simulink library "Sanu_Lib"  (R2025b)
settings: Solver=VariableStepAuto  StartTime=0.0  StopTime=10.0  RelTol=1e-3
libraries: simulink x16
settings Model: Creator=2503-00091  LastModifiedBy=2503-00091

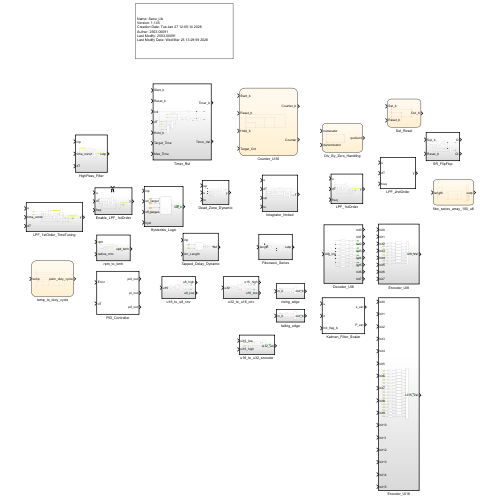
[thumbnail: Simulink's stored preview of the top-level diagram]
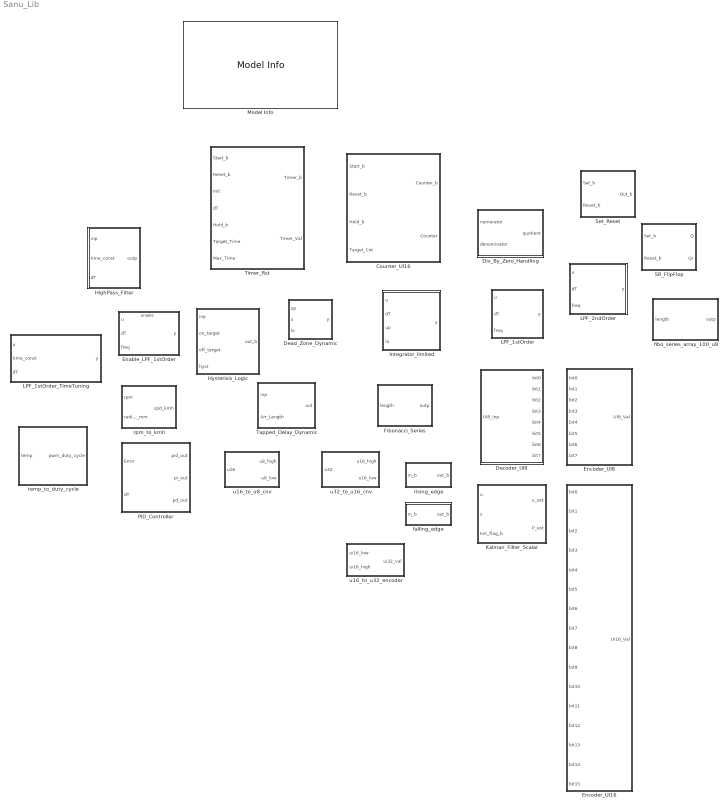
== system Sanu_Lib ==
  Counter_UI16 : Stateflow chart  TreatAsAtomicUnit=on  RTWFcnName=Counter_UI16  RTWFileName=Counter_UI16
      settings: RTWSystemCode=Reusable function  RTWFcnNameOpts=User specified  RTWFileNameOpts=User specified
  Dead_Zone_Dynamic : Subsystem  TreatAsAtomicUnit=on  RTWFcnName=Dead_Zone_Dynamic  RTWFileName=Dead_Zone_Dynamic
      settings: RTWFcnNameOpts=User specified  RTWFileNameOpts=User specified
  Decoder_UI8 : Subsystem  TreatAsAtomicUnit=on  RTWFcnName=Decoder_UI8  RTWFileName=Decoder_UI8
      settings: RTWFcnNameOpts=User specified  RTWFileNameOpts=User specified
  Div_By_Zero_Handling : Stateflow chart  TreatAsAtomicUnit=on  RTWFcnName=Div_By_Zero_Handling  RTWFileName=Div_By_Zero_Handling
      settings: RTWSystemCode=Reusable function  RTWFcnNameOpts=User specified  RTWFileNameOpts=User specified
  Enable_LPF_1stOrder : Subsystem  RTWFcnName=Enable_LPF_1stOrder  RTWFileName=Enable_LPF_1stOrder
      settings: RTWFcnNameOpts=User specified  RTWFileNameOpts=User specified
  Encoder_UI16 : Subsystem  TreatAsAtomicUnit=on  RTWFcnName=Encoder_UI16  RTWFileName=Encoder_UI16
      settings: RTWFcnNameOpts=User specified  RTWFileNameOpts=User specified
  Encoder_UI8 : Subsystem  TreatAsAtomicUnit=on  RTWFcnName=Encoder_UI8  RTWFileName=Encoder_UI8
      settings: RTWFcnNameOpts=User specified  RTWFileNameOpts=User specified
  Fibonacci_Series : Subsystem  TreatAsAtomicUnit=on  RTWFcnName=fibonacci_series_U8  RTWFileName=fibonacci_series_U8
      settings: RTWFcnNameOpts=User specified  RTWFileNameOpts=User specified
  HighPass_Filter : Subsystem  TreatAsAtomicUnit=on  RTWFcnName=HighPass_Filter  RTWFileName=HighPass_Filter
      settings: RTWFcnNameOpts=User specified  RTWFileNameOpts=User specified
  Hysterisis_Logic : Subsystem  TreatAsAtomicUnit=on  RTWFcnName=Hysterisis_Logic  RTWFileName=Hysterisis_Logic
      settings: RTWFcnNameOpts=User specified  RTWFileNameOpts=User specified
  Integrator_limited : Subsystem  TreatAsAtomicUnit=on  RTWFcnName=Integrator_limited  RTWFileName=Integrator_limited
      settings: RTWFcnNameOpts=User specified  RTWFileNameOpts=User specified
  Kalman_Filter_Scalar : Subsystem  TreatAsAtomicUnit=on  RTWFcnName=Kalman_Filter_Scalar  RTWFileName=Kalman_Filter_Scalar  mask{A_Gain=1, B_Gain=0, H_Gain=1, Q_Gain=0.01, R_Gain=0.1, x_est_init=0, P_est_init=1}
      settings: RTWFcnNameOpts=User specified  RTWFileNameOpts=User specified
      mask TypeOptions A_Gain: A_Gain/Value
      mask TypeOptions B_Gain: B_Gain/Gain
      mask TypeOptions H_Gain: H_Gain/Value
      mask TypeOptions Q_Gain: Q_Const/Value
      mask TypeOptions R_Gain: R_Const/Value
      mask TypeOptions x_est_init: x_init/Value
      mask TypeOptions P_est_init: P_init/Value
  LPF_1stOrder : Subsystem  TreatAsAtomicUnit=on  RTWFcnName=LPF_1stOrder  RTWFileName=LPF_1stOrder
      settings: RTWFcnNameOpts=User specified  RTWFileNameOpts=User specified
  LPF_1stOrder_TimeTuning : Subsystem  TreatAsAtomicUnit=on  RTWFcnName=LPF_1stOrder_TimeTuning  RTWFileName=LPF_1stOrder_TimeTuning
      settings: RTWFcnNameOpts=User specified  RTWFileNameOpts=User specified
  LPF_2ndOrder : Subsystem  TreatAsAtomicUnit=on  RTWFcnName=LPF_2ndOrder  RTWFileName=LPF_2ndOrder  mask{Gain=1}
      mask prompts: Gain "Damping_Coefficient:"
      settings: RTWFcnNameOpts=User specified  RTWFileNameOpts=User specified
      mask TypeOptions Gain: damping_coeff/Gain
  Model Info : simulink/Model-Wide Utilities/Model Info  Frame=on  DisplayStringWithTags=|  HorizontalTextAlignment=Left  LeftAlignmentValue=0.02
      | Name: %<ModelName>
      | Version: %<ModelVersion>
      | Creation Date: %<Created>
      | Author: %<Creator>
      | Last Modify: %<LastModifiedBy>
      | Last Modify Date: %<LastModificationDate>
  PID_Controller : Subsystem  TreatAsAtomicUnit=on  RTWFcnName=PID_Controller  RTWFileName=PID_Controller  mask{P_Gain=1, I_Gain=1, D_Gain=0, N_Gain=100}
      mask prompts: N_Gain "Filter(N)_Coeff:"
      settings: RTWFcnNameOpts=User specified  RTWFileNameOpts=User specified
      mask TypeOptions P_Gain: P_Gain/Gain
      mask TypeOptions I_Gain: I_Gain/Gain
      mask TypeOptions D_Gain: D_Gain/Gain
      mask TypeOptions N_Gain: N_Coeff/Gain
  SR_FlipFlop : Subsystem  TreatAsAtomicUnit=on  RTWFcnName=SR_FlipFlop  RTWFileName=SR_FlipFlop
      settings: RTWFcnNameOpts=User specified  RTWFileNameOpts=User specified
  Set_Reset : Stateflow chart  TreatAsAtomicUnit=on  RTWFcnName=Set_Reset  RTWFileName=Set_Reset
      settings: RTWSystemCode=Reusable function  RTWFcnNameOpts=User specified  RTWFileNameOpts=User specified
  Tapped_Delay_Dynamic : Subsystem  TreatAsAtomicUnit=on  RTWFcnName=Tapped_Delay_Dynamic  RTWFileName=Tapped_Delay_Dynamic
      settings: RTWFcnNameOpts=User specified  RTWFileNameOpts=User specified
  Timer_Rst : Subsystem  TreatAsAtomicUnit=on  RTWFcnName=Timer_Rst  RTWFileName=Timer_Rst
      settings: RTWFcnNameOpts=User specified  RTWFileNameOpts=User specified
  falling_edge : Subsystem  TreatAsAtomicUnit=on  RTWFcnName=falling_edge  RTWFileName=falling_edge
      settings: RTWFcnNameOpts=User specified  RTWFileNameOpts=User specified
  fibo_series_array_100_u8 : Stateflow chart  TreatAsAtomicUnit=on  RTWFcnName=fibo_series_array_100_u8  RTWFileName=fibo_series_array_100_u8
      settings: RTWSystemCode=Reusable function  RTWFcnNameOpts=User specified  RTWFileNameOpts=User specified
  rising_edge : Subsystem  TreatAsAtomicUnit=on  RTWFcnName=rising_edge  RTWFileName=rising_edge
      settings: RTWFcnNameOpts=User specified  RTWFileNameOpts=User specified
  rpm_to_kmh : Subsystem  TreatAsAtomicUnit=on  RTWFcnName=rpm_to_kmph  RTWFileName=rpm_to_kmph
      settings: RTWFcnNameOpts=User specified  RTWFileNameOpts=User specified
  temp_to_duty_cycle : Stateflow chart  TreatAsAtomicUnit=on  RTWFcnName=temp_to_duty_cycle  RTWFileName=temp_to_duty_cycle
      settings: RTWSystemCode=Reusable function  RTWFcnNameOpts=User specified  RTWFileNameOpts=User specified
  u16_to_u32_encoder : Subsystem  TreatAsAtomicUnit=on  RTWFcnName=u16_to_u32_encoder  RTWFileName=u16_to_u32_encoder
      settings: RTWFcnNameOpts=User specified  RTWFileNameOpts=User specified
  u16_to_u8_cnv : Subsystem  TreatAsAtomicUnit=on  RTWFcnName=u16_to_u8  RTWFileName=u16_to_u8
      settings: RTWFcnNameOpts=User specified  RTWFileNameOpts=User specified
  u32_to_u16_cnv : Subsystem  TreatAsAtomicUnit=on  RTWFcnName=u32_to_u16  RTWFileName=u32_to_u16
      settings: RTWFcnNameOpts=User specified  RTWFileNameOpts=User specified

== system Sanu_Lib/Dead_Zone_Dynamic ==
  up : Inport
  u : Inport  Port=2
  lo : Inport  Port=3
  Relational Operator : RelationalOperator  OutDataTypeStr=boolean  RndMeth=Simplest  InputSameDT=off
  Relational Operator1 : RelationalOperator  Operator=>  OutDataTypeStr=boolean  RndMeth=Simplest  InputSameDT=off
  Subtract : Sum  Inputs=+-
  Switch : Switch  Criteria=u2 ~= 0  SaturateOnIntegerOverflow=off  InputSameDT=off
  Switch1 : Switch  Criteria=u2 ~= 0  SaturateOnIntegerOverflow=off  InputSameDT=off
  y : Outport
  wires:
  up/1 -> Relational Operator/2, Switch/1
  u/1 -> Subtract/1, Relational Operator/1, Switch1/1, Relational Operator1/1
  Relational Operator/1 -> Switch/2
  Relational Operator1/1 -> Switch1/2
  lo/1 -> Switch1/3, Relational Operator1/2
  Switch1/1 -> Switch/3
  Subtract/1 -> y/1
  Switch/1 -> Subtract/2

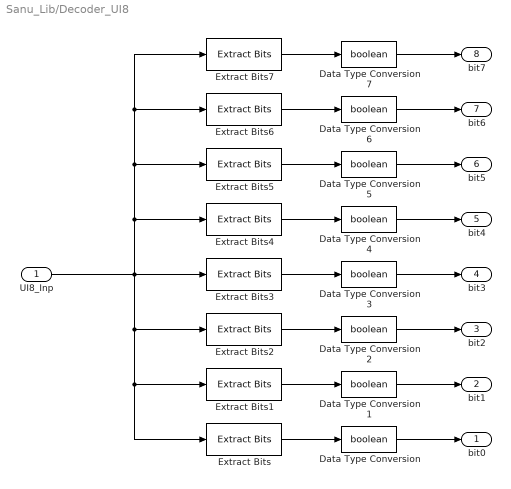
== system Sanu_Lib/Decoder_UI8 ==
  UI8_Inp : Inport  OutDataTypeStr=uint8
  Data Type Conversion{,1..7} (8 alike) : DataTypeConversion  OutDataTypeStr=boolean  SaturateOnIntegerOverflow=off  RndMeth=Floor
  Extract Bits : simulink/Logic and Bit Operations/Extract Bits  bitsToExtract=Range of bits  numBits=8  bitIdxRange=[0 0]  outScalingMode=Preserve fixed-point scaling
  Extract Bits1 : simulink/Logic and Bit Operations/Extract Bits  bitsToExtract=Range of bits  numBits=8  bitIdxRange=[1 1]  outScalingMode=Preserve fixed-point scaling
  Extract Bits2 : simulink/Logic and Bit Operations/Extract Bits  bitsToExtract=Range of bits  numBits=8  bitIdxRange=[2 2]  outScalingMode=Preserve fixed-point scaling
  Extract Bits3 : simulink/Logic and Bit Operations/Extract Bits  bitsToExtract=Range of bits  numBits=8  bitIdxRange=[3 3]  outScalingMode=Preserve fixed-point scaling
  Extract Bits4 : simulink/Logic and Bit Operations/Extract Bits  bitsToExtract=Range of bits  numBits=8  bitIdxRange=[4 4]  outScalingMode=Preserve fixed-point scaling
  Extract Bits5 : simulink/Logic and Bit Operations/Extract Bits  bitsToExtract=Range of bits  numBits=8  bitIdxRange=[5 5]  outScalingMode=Preserve fixed-point scaling
  Extract Bits6 : simulink/Logic and Bit Operations/Extract Bits  bitsToExtract=Range of bits  numBits=8  bitIdxRange=[6 6]  outScalingMode=Preserve fixed-point scaling
  Extract Bits7 : simulink/Logic and Bit Operations/Extract Bits  bitsToExtract=Range of bits  numBits=8  bitIdxRange=[7 7]  outScalingMode=Preserve fixed-point scaling
  bit0 : Outport
  bit1 : Outport  Port=2
  bit2 : Outport  Port=3
  bit3 : Outport  Port=4
  bit4 : Outport  Port=5
  bit5 : Outport  Port=6
  bit6 : Outport  Port=7
  bit7 : Outport  Port=8
  wires:
  UI8_Inp/1 -> Extract Bits5/1, Extract Bits6/1, Extract Bits7/1, Extract Bits4/1, Extract Bits3/1, Extract Bits2/1, Extract Bits1/1, Extract Bits/1
  Extract Bits/1 -> Data Type Conversion/1
  Data Type Conversion/1 -> bit0/1
  Data Type Conversion1/1 -> bit1/1
  Data Type Conversion3/1 -> bit3/1
  Data Type Conversion2/1 -> bit2/1
  Data Type Conversion4/1 -> bit4/1
  Data Type Conversion5/1 -> bit5/1
  Data Type Conversion7/1 -> bit7/1
  Data Type Conversion6/1 -> bit6/1
  Extract Bits1/1 -> Data Type Conversion1/1
  Extract Bits2/1 -> Data Type Conversion2/1
  Extract Bits3/1 -> Data Type Conversion3/1
  Extract Bits4/1 -> Data Type Conversion4/1
  Extract Bits5/1 -> Data Type Conversion5/1
  Extract Bits6/1 -> Data Type Conversion6/1
  Extract Bits7/1 -> Data Type Conversion7/1

== system Sanu_Lib/Enable_LPF_1stOrder ==
  note: y(t) = y(t-1) + (u(t) - y(t-1)) * dT * freq
  u : Inport
  dT : Inport  Port=2
  freq : Inport  Port=3
  Enable : EnablePort  StatesWhenEnabling=reset
  Product : Product
  Product1 : Product
  Substract : Sum  Inputs=+-
  delay_y : UnitDelay  SampleTime=-1  HasFrameUpgradeWarning=on
      settings: AttributesFormatString=Init: %<InitialCondition>
  lpf_out : Sum
  y : Outport
  wires:
  Product1/1 -> lpf_out/1
  freq/1 -> Product1/1
  lpf_out/1 -> delay_y/1, y/1
  u/1 -> Substract/1
  Product/1 -> Product1/2
  Substract/1 -> Product/2
  dT/1 -> Product/1
  delay_y/1 -> Substract/2, lpf_out/2

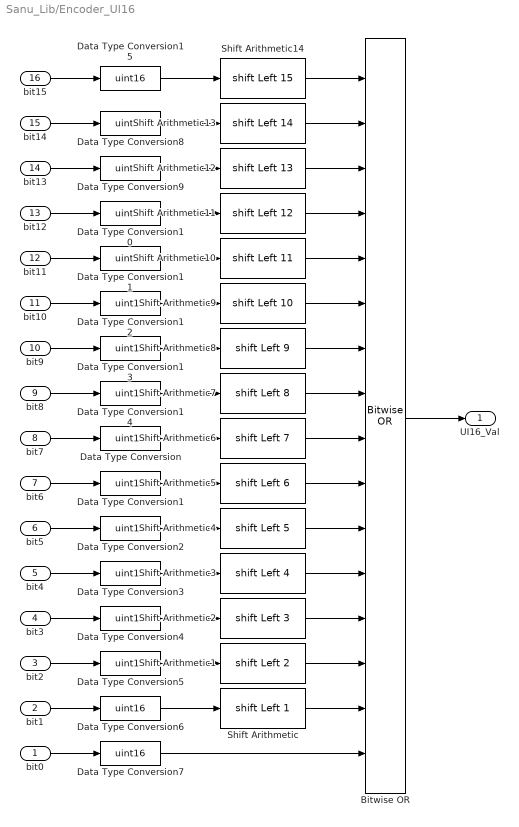
== system Sanu_Lib/Encoder_UI16 ==
  bit0 : Inport  OutDataTypeStr=boolean
  bit1 : Inport  Port=2  OutDataTypeStr=boolean
  bit2 : Inport  Port=3  OutDataTypeStr=boolean
  bit3 : Inport  Port=4  OutDataTypeStr=boolean
  bit4 : Inport  Port=5  OutDataTypeStr=boolean
  bit5 : Inport  Port=6  OutDataTypeStr=boolean
  bit6 : Inport  Port=7  OutDataTypeStr=boolean
  bit7 : Inport  Port=8  OutDataTypeStr=boolean
  bit8 : Inport  Port=9  OutDataTypeStr=boolean
  bit9 : Inport  Port=10  OutDataTypeStr=boolean
  bit10 : Inport  Port=11  OutDataTypeStr=boolean
  bit11 : Inport  Port=12  OutDataTypeStr=boolean
  bit12 : Inport  Port=13  OutDataTypeStr=boolean
  bit13 : Inport  Port=14  OutDataTypeStr=boolean
  bit14 : Inport  Port=15  OutDataTypeStr=boolean
  bit15 : Inport  Port=16  OutDataTypeStr=boolean
  Bitwise OR : simulink/Logic and Bit Operations/Bitwise Operator  logicop=OR  UseBitMask=off  NumInputPorts=16  BitMask=bin2dec('11011001')  BitMaskRealWorld=Stored Integer
      settings: LibrarySourceBlock=|
      | simulink/Quick Insert/Logic and Bit
      | Operations/Bitwise OR
  Data Type Conversion{,1..15} (16 alike) : DataTypeConversion  OutDataTypeStr=uint16  SaturateOnIntegerOverflow=off  RndMeth=Floor
  Shift Arithmetic : ArithShift  BitShiftNumber=1  BitShiftDirection=Left
  Shift Arithmetic1 : ArithShift  BitShiftNumber=2  BitShiftDirection=Left
  Shift Arithmetic10 : ArithShift  BitShiftNumber=11  BitShiftDirection=Left
  Shift Arithmetic11 : ArithShift  BitShiftNumber=12  BitShiftDirection=Left
  Shift Arithmetic12 : ArithShift  BitShiftNumber=13  BitShiftDirection=Left
  Shift Arithmetic13 : ArithShift  BitShiftNumber=14  BitShiftDirection=Left
  Shift Arithmetic14 : ArithShift  BitShiftNumber=15  BitShiftDirection=Left
  Shift Arithmetic2 : ArithShift  BitShiftNumber=3  BitShiftDirection=Left
  Shift Arithmetic3 : ArithShift  BitShiftNumber=4  BitShiftDirection=Left
  Shift Arithmetic4 : ArithShift  BitShiftNumber=5  BitShiftDirection=Left
  Shift Arithmetic5 : ArithShift  BitShiftNumber=6  BitShiftDirection=Left
  Shift Arithmetic6 : ArithShift  BitShiftNumber=7  BitShiftDirection=Left
  Shift Arithmetic7 : ArithShift  BitShiftNumber=8  BitShiftDirection=Left
  Shift Arithmetic8 : ArithShift  BitShiftNumber=9  BitShiftDirection=Left
  Shift Arithmetic9 : ArithShift  BitShiftNumber=10  BitShiftDirection=Left
  UI16_Val : Outport
  wires:
  bit7/1 -> Data Type Conversion/1
  bit2/1 -> Data Type Conversion5/1
  bit5/1 -> Data Type Conversion2/1
  Data Type Conversion1/1 -> Shift Arithmetic5/1
  Data Type Conversion2/1 -> Shift Arithmetic4/1
  Data Type Conversion4/1 -> Shift Arithmetic2/1
  bit0/1 -> Data Type Conversion7/1
  Data Type Conversion3/1 -> Shift Arithmetic3/1
  bit3/1 -> Data Type Conversion4/1
  Bitwise OR/1 -> UI16_Val/1
  Data Type Conversion6/1 -> Shift Arithmetic/1
  Data Type Conversion5/1 -> Shift Arithmetic1/1
  bit6/1 -> Data Type Conversion1/1
  Data Type Conversion/1 -> Shift Arithmetic6/1
  bit1/1 -> Data Type Conversion6/1
  bit4/1 -> Data Type Conversion3/1
  Shift Arithmetic1/1 -> Bitwise OR/14
  Shift Arithmetic/1 -> Bitwise OR/15
  Shift Arithmetic2/1 -> Bitwise OR/13
  Data Type Conversion7/1 -> Bitwise OR/16
  Shift Arithmetic3/1 -> Bitwise OR/12
  bit11/1 -> Data Type Conversion11/1
  bit8/1 -> Data Type Conversion14/1
  Data Type Conversion8/1 -> Shift Arithmetic13/1
  bit13/1 -> Data Type Conversion9/1
  Data Type Conversion13/1 -> Shift Arithmetic8/1
  Data Type Conversion14/1 -> Shift Arithmetic7/1
  bit10/1 -> Data Type Conversion12/1
  Data Type Conversion11/1 -> Shift Arithmetic10/1
  Data Type Conversion12/1 -> Shift Arithmetic9/1
  Data Type Conversion10/1 -> Shift Arithmetic11/1
  Data Type Conversion9/1 -> Shift Arithmetic12/1
  bit12/1 -> Data Type Conversion10/1
  bit9/1 -> Data Type Conversion13/1
  bit14/1 -> Data Type Conversion8/1
  bit15/1 -> Data Type Conversion15/1
  Data Type Conversion15/1 -> Shift Arithmetic14/1
  Shift Arithmetic14/1 -> Bitwise OR/1
  Shift Arithmetic6/1 -> Bitwise OR/9
  Shift Arithmetic5/1 -> Bitwise OR/10
  Shift Arithmetic4/1 -> Bitwise OR/11
  Shift Arithmetic13/1 -> Bitwise OR/2
  Shift Arithmetic12/1 -> Bitwise OR/3
  Shift Arithmetic11/1 -> Bitwise OR/4
  Shift Arithmetic10/1 -> Bitwise OR/5
  Shift Arithmetic9/1 -> Bitwise OR/6
  Shift Arithmetic8/1 -> Bitwise OR/7
  Shift Arithmetic7/1 -> Bitwise OR/8

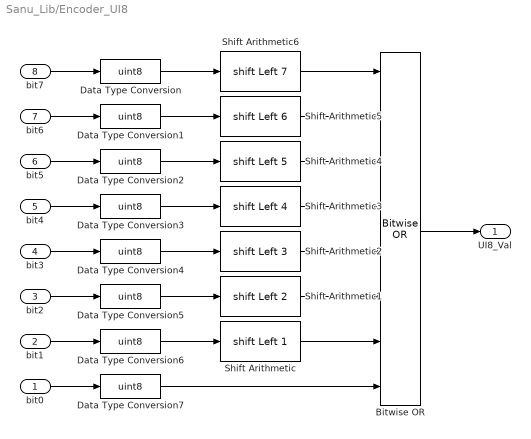
== system Sanu_Lib/Encoder_UI8 ==
  bit0 : Inport  OutDataTypeStr=boolean
  bit1 : Inport  Port=2  OutDataTypeStr=boolean
  bit2 : Inport  Port=3  OutDataTypeStr=boolean
  bit3 : Inport  Port=4  OutDataTypeStr=boolean
  bit4 : Inport  Port=5  OutDataTypeStr=boolean
  bit5 : Inport  Port=6  OutDataTypeStr=boolean
  bit6 : Inport  Port=7  OutDataTypeStr=boolean
  bit7 : Inport  Port=8  OutDataTypeStr=boolean
  Bitwise OR : simulink/Logic and Bit Operations/Bitwise Operator  logicop=OR  UseBitMask=off  NumInputPorts=8  BitMask=bin2dec('11011001')  BitMaskRealWorld=Stored Integer
      settings: LibrarySourceBlock=|
      | simulink/Quick Insert/Logic and Bit
      | Operations/Bitwise OR
  Data Type Conversion{,1..7} (8 alike) : DataTypeConversion  OutDataTypeStr=uint8  SaturateOnIntegerOverflow=off  RndMeth=Floor
  Shift Arithmetic : ArithShift  BitShiftNumber=1  BitShiftDirection=Left
  Shift Arithmetic1 : ArithShift  BitShiftNumber=2  BitShiftDirection=Left
  Shift Arithmetic2 : ArithShift  BitShiftNumber=3  BitShiftDirection=Left
  Shift Arithmetic3 : ArithShift  BitShiftNumber=4  BitShiftDirection=Left
  Shift Arithmetic4 : ArithShift  BitShiftNumber=5  BitShiftDirection=Left
  Shift Arithmetic5 : ArithShift  BitShiftNumber=6  BitShiftDirection=Left
  Shift Arithmetic6 : ArithShift  BitShiftNumber=7  BitShiftDirection=Left
  UI8_Val : Outport
  wires:
  bit1/1 -> Data Type Conversion6/1
  Shift Arithmetic/1 -> Bitwise OR/7
  bit0/1 -> Data Type Conversion7/1
  Shift Arithmetic1/1 -> Bitwise OR/6
  bit2/1 -> Data Type Conversion5/1
  bit4/1 -> Data Type Conversion3/1
  bit3/1 -> Data Type Conversion4/1
  bit5/1 -> Data Type Conversion2/1
  bit6/1 -> Data Type Conversion1/1
  bit7/1 -> Data Type Conversion/1
  Shift Arithmetic6/1 -> Bitwise OR/1
  Shift Arithmetic5/1 -> Bitwise OR/2
  Shift Arithmetic4/1 -> Bitwise OR/3
  Shift Arithmetic3/1 -> Bitwise OR/4
  Shift Arithmetic2/1 -> Bitwise OR/5
  Bitwise OR/1 -> UI8_Val/1
  Data Type Conversion/1 -> Shift Arithmetic6/1
  Data Type Conversion1/1 -> Shift Arithmetic5/1
  Data Type Conversion2/1 -> Shift Arithmetic4/1
  Data Type Conversion3/1 -> Shift Arithmetic3/1
  Data Type Conversion4/1 -> Shift Arithmetic2/1
  Data Type Conversion5/1 -> Shift Arithmetic1/1
  Data Type Conversion6/1 -> Shift Arithmetic/1
  Data Type Conversion7/1 -> Bitwise OR/8

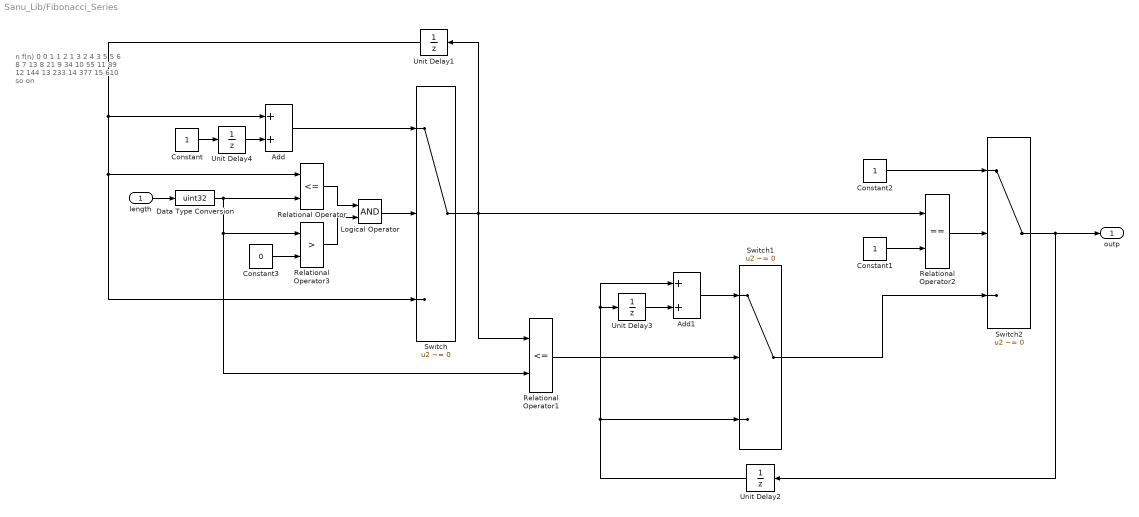
== system Sanu_Lib/Fibonacci_Series ==
  note: n f(n)
      |
      | 0 0
      | 1 1
      | 2 1
      | 3 2
      | 4 3
      | 5 5
      | 6 8
      | 7 13
      | 8 21
      | 9 34
      | 10 55
      | 11 89
      | 12 144
      | 13 233
      | 14 377
      | 15 610
      | so on
  length : Inport
  Add : Sum
  Add1 : Sum  OutDataTypeStr=single
  Constant : Constant  OutDataTypeStr=uint32  SampleTime=-1
  Constant1 : Constant  OutDataTypeStr=uint32  SampleTime=-1
  Constant2 : Constant  OutDataTypeStr=single  SampleTime=-1
  Constant3 : Constant  Value=0  OutDataTypeStr=uint32  SampleTime=-1
  Data Type Conversion : DataTypeConversion  OutDataTypeStr=uint32  SaturateOnIntegerOverflow=off  RndMeth=Floor
  Logical Operator : Logic  AllPortsSameDT=off  OutDataTypeStr=boolean
  Relational Operator : RelationalOperator  Operator=<=  OutDataTypeStr=boolean  RndMeth=Simplest  InputSameDT=off
  Relational Operator1 : RelationalOperator  Operator=<=  OutDataTypeStr=boolean  RndMeth=Simplest  InputSameDT=off
  Relational Operator2 : RelationalOperator  Operator===  OutDataTypeStr=boolean  RndMeth=Simplest  InputSameDT=off
  Relational Operator3 : RelationalOperator  Operator=>  OutDataTypeStr=boolean  RndMeth=Simplest  InputSameDT=off
  Switch : Switch  Criteria=u2 ~= 0  SaturateOnIntegerOverflow=off  InputSameDT=off
  Switch1 : Switch  Criteria=u2 ~= 0  SaturateOnIntegerOverflow=off  InputSameDT=off
  Switch2 : Switch  Criteria=u2 ~= 0  SaturateOnIntegerOverflow=off  InputSameDT=off
  Unit Delay{1..4} (4 alike) : UnitDelay  SampleTime=-1  HasFrameUpgradeWarning=on
      settings: AttributesFormatString=Init: %<InitialCondition>
  outp : Outport
  wires:
  Relational Operator2/1 -> Switch2/2
  Constant1/1 -> Relational Operator2/2
  Unit Delay1/1 -> Switch/3, Relational Operator/1, Add/1
  Constant/1 -> Unit Delay4/1
  Switch/1 -> Unit Delay1/1, Relational Operator2/1, Relational Operator1/1
  Add/1 -> Switch/1
  Constant2/1 -> Switch2/1
  Relational Operator/1 -> Logical Operator/1
  Unit Delay2/1 -> Add1/1, Unit Delay3/1, Switch1/3
  Add1/1 -> Switch1/1
  Relational Operator1/1 -> Switch1/2
  Unit Delay3/1 -> Add1/2
  length/1 -> Data Type Conversion/1
  Switch1/1 -> Switch2/3
  Switch2/1 -> Unit Delay2/1, outp/1
  Unit Delay4/1 -> Add/2
  Data Type Conversion/1 -> Relational Operator/2, Relational Operator3/1, Relational Operator1/2
  Constant3/1 -> Relational Operator3/2
  Relational Operator3/1 -> Logical Operator/2
  Logical Operator/1 -> Switch/2

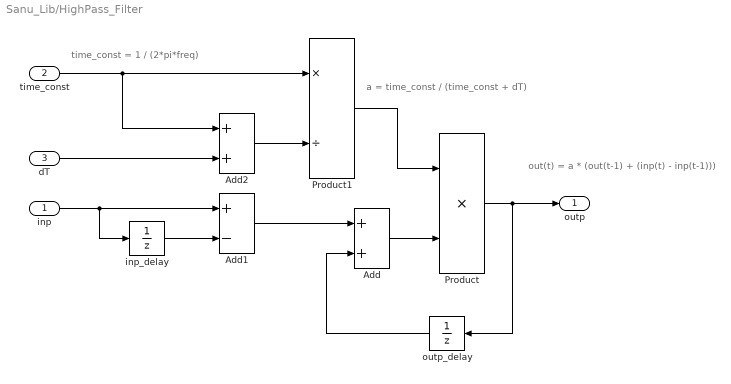
== system Sanu_Lib/HighPass_Filter ==
  note: out(t) = a * (out(t-1) + (inp(t) - inp(t-1)))
  note: time_const = 1 / (2*pi*freq)
  note: a = time_const / (time_const + dT)
  inp : Inport
  time_const : Inport  Port=2
  dT : Inport  Port=3
  Add : Sum
  Add1 : Sum  Inputs=+-
  Add2 : Sum  Inputs=2
  Product : Product
  Product1 : Product  Inputs=*/
  inp_delay : UnitDelay  SampleTime=-1  HasFrameUpgradeWarning=on
      settings: AttributesFormatString=Init: %<InitialCondition>
  outp_delay : UnitDelay  SampleTime=-1  HasFrameUpgradeWarning=on
      settings: AttributesFormatString=Init: %<InitialCondition>
  outp : Outport
  wires:
  outp_delay/1 -> Add/2
  inp/1 -> inp_delay/1, Add1/1
  inp_delay/1 -> Add1/2
  Add1/1 -> Add/1
  Add/1 -> Product/2
  Product/1 -> outp_delay/1, outp/1
  Add2/1 -> Product1/2
  dT/1 -> Add2/2
  time_const/1 -> Add2/1, Product1/1
  Product1/1 -> Product/1

== system Sanu_Lib/Hysterisis_Logic ==
  inp : Inport
  on_target : Inport  Port=2
  off_target : Inport  Port=3
  hyst : Inport  Port=4
  Hysterisis : Stateflow chart  TreatAsAtomicUnit=on
  out_b : Outport
  wires:
  on_target/1 -> Hysterisis/2(on_target)
  hyst/1 -> Hysterisis/4(hyst)
  inp/1 -> Hysterisis/1(inp)
  Hysterisis/1(out_b) -> out_b/1
  off_target/1 -> Hysterisis/3(off_target)

== system Sanu_Lib/Integrator_limited ==
  u : Inport
  dT : Inport  Port=2
  up : Inport  Port=3
  lo : Inport  Port=4
  Add : Sum
  Max : MinMax  Function=max  Inputs=2
  Min : MinMax  Inputs=2
  Product : Product
  integrator_dly : UnitDelay  SampleTime=-1  HasFrameUpgradeWarning=on
      settings: AttributesFormatString=Init: %<InitialCondition>
  y : Outport
  wires:
  u/1 -> Product/1
  dT/1 -> Product/2
  Product/1 -> Add/2
  Add/1 -> Min/1
  up/1 -> Min/2
  Max/1 -> integrator_dly/1, y/1
  Min/1 -> Max/1
  lo/1 -> Max/2
  integrator_dly/1 -> Add/1

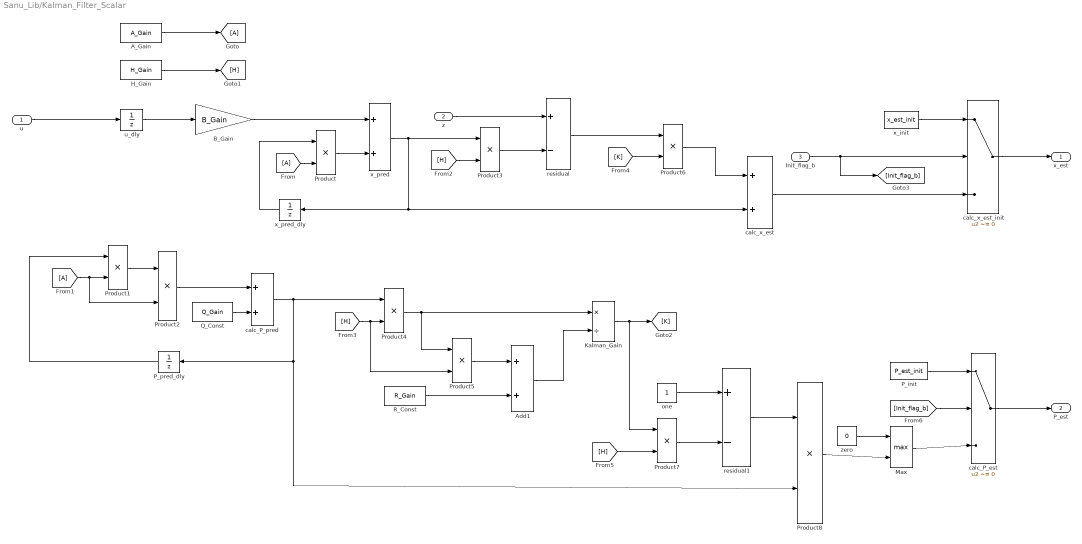
== system Sanu_Lib/Kalman_Filter_Scalar ==
  u : Inport
  z : Inport  Port=2
  Init_flag_b : Inport  Port=3
  A_Gain : Constant  Value=A_Gain  OutDataTypeStr=single  SampleTime=-1
  Add1 : Sum
  B_Gain : Gain  Gain=B_Gain
  From : From
  From1 : From
  Goto : Goto
  H_Gain : Constant  Value=H_Gain  OutDataTypeStr=single  SampleTime=-1
  Kalman_Gain : Product  Inputs=*/
  Max : MinMax  Function=max  Inputs=2
  P_init : Constant  Value=P_est_init  OutDataTypeStr=single  SampleTime=-1
  P_pred_dly : UnitDelay  SampleTime=-1  HasFrameUpgradeWarning=on
      settings: AttributesFormatString=Init: %<InitialCondition>
  Product{,1..8} (9 alike) : Product
  Q_Const : Constant  Value=Q_Gain  OutDataTypeStr=single  SampleTime=-1
  R_Const : Constant  Value=R_Gain  OutDataTypeStr=single  SampleTime=-1
  calc_P_est : Switch  Criteria=u2 ~= 0  SaturateOnIntegerOverflow=off  InputSameDT=off
  calc_P_pred : Sum
  calc_x_est : Sum  Inputs=2
  calc_x_est_init : Switch  Criteria=u2 ~= 0  SaturateOnIntegerOverflow=off  InputSameDT=off
  one : Constant  OutDataTypeStr=single  SampleTime=-1
  residual : Sum  Inputs=+-
  residual1 : Sum  Inputs=+-
  u_dly : UnitDelay  SampleTime=-1  HasFrameUpgradeWarning=on
      settings: AttributesFormatString=Init: %<InitialCondition>
  x_init : Constant  Value=x_est_init  OutDataTypeStr=single  SampleTime=-1
  x_pred : Sum
  x_pred_dly : UnitDelay  SampleTime=-1  HasFrameUpgradeWarning=on
      settings: AttributesFormatString=Init: %<InitialCondition>
  zero : Constant  Value=0  OutDataTypeStr=single  SampleTime=-1
  x_est : Outport
  P_est : Outport  Port=2
  wires:
  x_pred_dly/1 -> Product/1
  u/1 -> u_dly/1
  B_Gain/1 -> x_pred/1
  Product/1 -> x_pred/2
  u_dly/1 -> B_Gain/1
  x_pred/1 -> Product3/1, x_pred_dly/1, calc_x_est/2
  A_Gain/1 -> Goto/1
  From/1 -> Product/2
  P_pred_dly/1 -> Product1/1
  From1/1 -> Product2/2, Product1/2
  Product1/1 -> Product2/1
  Product2/1 -> calc_P_pred/1
  Q_Const/1 -> calc_P_pred/2
  Product3/1 -> residual/2
  z/1 -> residual/1
  residual/1 -> Product6/1
  Product6/1 -> calc_x_est/1
  H_Gain/1 -> [H]
  [H] -> Product3/2
  [H] -> Product5/2, Product4/2
  Product4/1 -> Kalman_Gain/1, Product5/1
  Product5/1 -> Add1/1
  R_Const/1 -> Add1/2
  Add1/1 -> Kalman_Gain/2
  Kalman_Gain/1 -> Product7/1, [K]
  [K] -> Product6/2
  calc_P_pred/1 -> P_pred_dly/1, Product8/2, Product4/1
  calc_x_est_init/1 -> x_est/1
  one/1 -> residual1/1
  Product7/1 -> residual1/2
  [H] -> Product7/2
  residual1/1 -> Product8/1
  [Init_flag_b] -> calc_P_est/2
  Max/1 -> calc_P_est/3
  calc_P_est/1 -> P_est/1
  Product8/1 -> Max/2
  Init_flag_b/1 -> calc_x_est_init/2, [Init_flag_b]
  zero/1 -> Max/1
  x_init/1 -> calc_x_est_init/1
  calc_x_est/1 -> calc_x_est_init/3
  P_init/1 -> calc_P_est/1

== system Sanu_Lib/LPF_1stOrder ==
  note: y(t) = y(t-1) + (u(t) - y(t-1)) * dT * freq
  u : Inport
  dT : Inport  Port=2
  freq : Inport  Port=3
  Product : Product
  Product1 : Product
  Substract : Sum  Inputs=+-
  delay_y : UnitDelay  SampleTime=-1  HasFrameUpgradeWarning=on
      settings: AttributesFormatString=Init: %<InitialCondition>
  lpf_out : Sum
  y : Outport
  wires:
  lpf_out/1 -> delay_y/1, y/1
  delay_y/1 -> Substract/2, lpf_out/2
  u/1 -> Substract/1
  Substract/1 -> Product/2
  dT/1 -> Product/1
  Product/1 -> Product1/2
  Product1/1 -> lpf_out/1
  freq/1 -> Product1/1

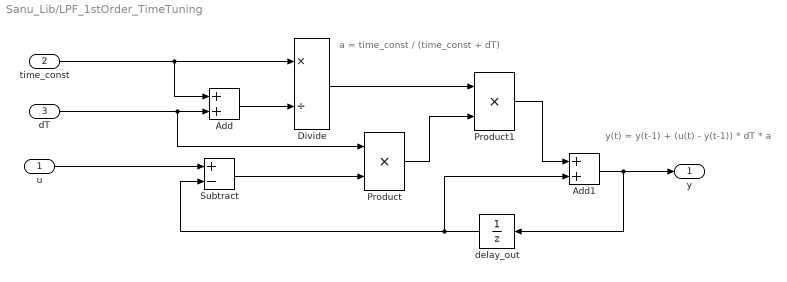
== system Sanu_Lib/LPF_1stOrder_TimeTuning ==
  note: a = time_const / (time_const + dT)
  note: y(t) = y(t-1) + (u(t) - y(t-1)) * dT * a
  u : Inport
  time_const : Inport  Port=2
  dT : Inport  Port=3
  Add : Sum
  Add1 : Sum
  Divide : Product  Inputs=*/
  Product : Product
  Product1 : Product
  Subtract : Sum  Inputs=+-
  delay_out : UnitDelay  SampleTime=-1  HasFrameUpgradeWarning=on
      settings: AttributesFormatString=Init: %<InitialCondition>
  y : Outport
  wires:
  time_const/1 -> Add/1, Divide/1
  dT/1 -> Product/1, Add/2
  Add/1 -> Divide/2
  delay_out/1 -> Subtract/2, Add1/2
  u/1 -> Subtract/1
  Subtract/1 -> Product/2
  Product/1 -> Product1/2
  Divide/1 -> Product1/1
  Product1/1 -> Add1/1
  Add1/1 -> y/1, delay_out/1

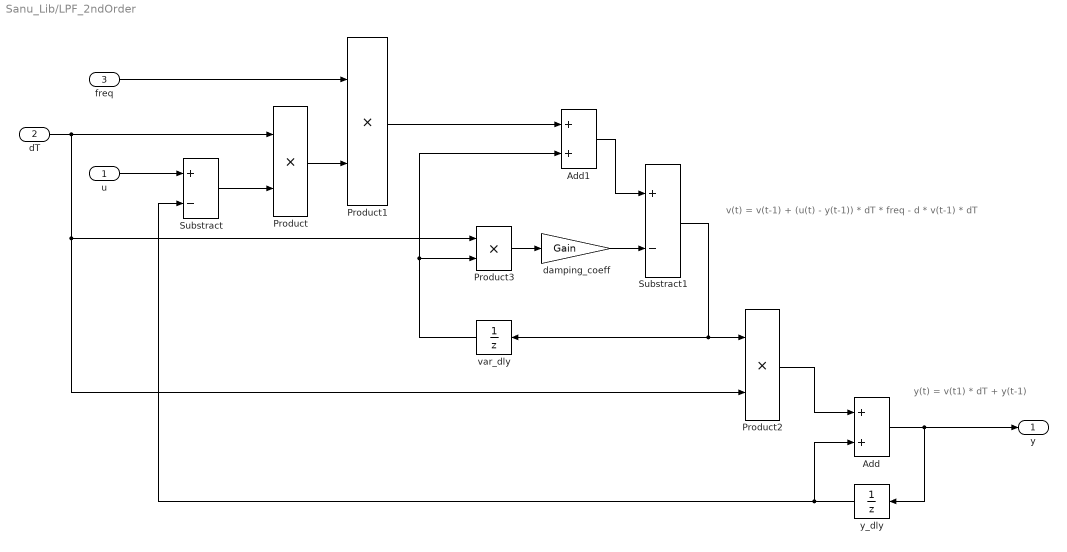
== system Sanu_Lib/LPF_2ndOrder ==
  note: y(t) = v(t1) * dT + y(t-1)
  note: v(t) = v(t-1) + (u(t) - y(t-1)) * dT * freq - d * v(t-1) * dT
  u : Inport
  dT : Inport  Port=2
  freq : Inport  Port=3
  Add : Sum  Inputs=2
  Add1 : Sum  Inputs=2
  Product{,1..3} (4 alike) : Product
  Substract : Sum  Inputs=+-
  Substract1 : Sum  Inputs=+-
  damping_coeff : Gain  Gain=Gain
  var_dly : UnitDelay  SampleTime=-1  HasFrameUpgradeWarning=on
      settings: AttributesFormatString=Init: %<InitialCondition>
  y_dly : UnitDelay  SampleTime=-1  HasFrameUpgradeWarning=on
      settings: AttributesFormatString=Init: %<InitialCondition>
  y : Outport
  wires:
  y_dly/1 -> Substract/2, Add/2
  u/1 -> Substract/1
  Add/1 -> y_dly/1, y/1
  Substract/1 -> Product/2
  freq/1 -> Product1/1
  Product/1 -> Product1/2
  dT/1 -> Product/1, Product2/2, Product3/1
  Product1/1 -> Add1/1
  var_dly/1 -> Add1/2, Product3/2
  Substract1/1 -> var_dly/1, Product2/1
  Product3/1 -> damping_coeff/1
  Product2/1 -> Add/1
  Add1/1 -> Substract1/1
  damping_coeff/1 -> Substract1/2

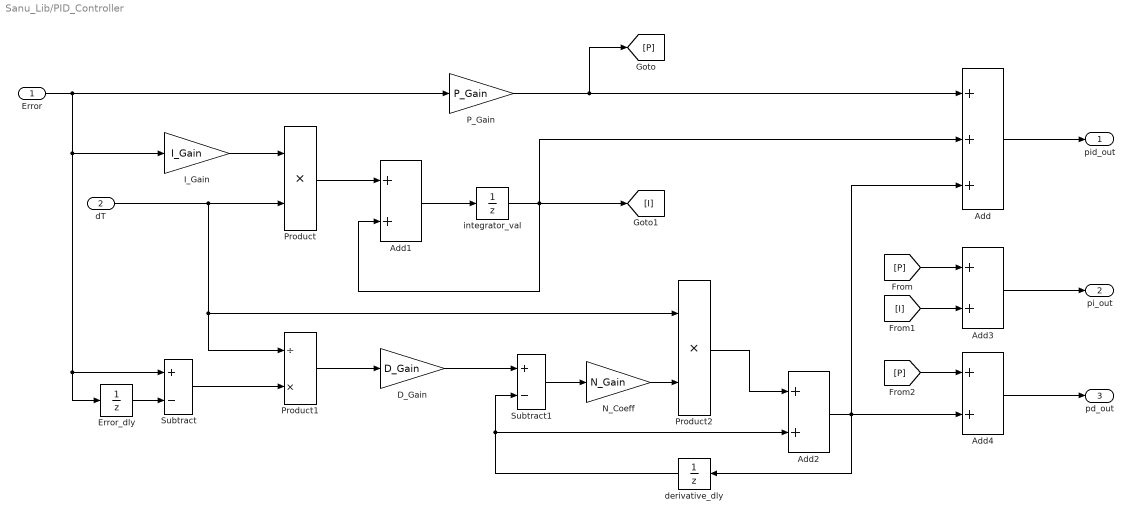
== system Sanu_Lib/PID_Controller ==
  Error : Inport
  dT : Inport  Port=2
  Add : Sum  Inputs=3
  Add{1..4} (4 alike) : Sum  Inputs=2
  D_Gain : Gain  Gain=D_Gain
  Error_dly : UnitDelay  SampleTime=-1  HasFrameUpgradeWarning=on
      settings: AttributesFormatString=Init: %<InitialCondition>
  I_Gain : Gain  Gain=I_Gain
  N_Coeff : Gain  Gain=N_Gain
  P_Gain : Gain  Gain=P_Gain
  Product : Product
  Product1 : Product  Inputs=/*
  Product2 : Product
  Subtract : Sum  Inputs=+-
  Subtract1 : Sum  Inputs=+-
  derivative_dly : UnitDelay  SampleTime=-1  HasFrameUpgradeWarning=on
      settings: AttributesFormatString=Init: %<InitialCondition>
  integrator_val : UnitDelay  SampleTime=-1  HasFrameUpgradeWarning=on
      settings: AttributesFormatString=Init: %<InitialCondition>
  pid_out : Outport
  pi_out : Outport  Port=2
  pd_out : Outport  Port=3
  wires:
  Error/1 -> Subtract/1, Error_dly/1, I_Gain/1, P_Gain/1
  P_Gain/1 -> [P], Add/1
  I_Gain/1 -> Product/1
  dT/1 -> Product/2, Product1/1, Product2/1
  Product/1 -> Add1/1
  Add1/1 -> integrator_val/1
  integrator_val/1 -> [I], Add1/2, Add/2
  Error_dly/1 -> Subtract/2
  Subtract/1 -> Product1/2
  Product1/1 -> D_Gain/1
  derivative_dly/1 -> Subtract1/2, Add2/2
  D_Gain/1 -> Subtract1/1
  Subtract1/1 -> N_Coeff/1
  N_Coeff/1 -> Product2/2
  Add2/1 -> Add/3, Add4/2, derivative_dly/1
  Add/1 -> pid_out/1
  [P] -> Add3/1
  [I] -> Add3/2
  Add3/1 -> pi_out/1
  [P] -> Add4/1
  Add4/1 -> pd_out/1
  Product2/1 -> Add2/1

== system Sanu_Lib/SR_FlipFlop ==
  Set_b : Inport
  Reset_b : Inport  Port=2
  Logical Operator : Logic  AllPortsSameDT=off  OutDataTypeStr=boolean
  Logical Operator1 : Logic  Operator=NOT  AllPortsSameDT=off  OutDataTypeStr=boolean
  Logical Operator2 : Logic  Operator=OR  AllPortsSameDT=off  OutDataTypeStr=boolean
  Logical Operator3 : Logic  Operator=NOR  AllPortsSameDT=off  OutDataTypeStr=boolean
  Q_dly : UnitDelay  SampleTime=-1  HasFrameUpgradeWarning=on
      settings: AttributesFormatString=Init: %<InitialCondition>
  Q : Outport
  Q! : Outport  Port=2
  wires:
  Logical Operator1/1 -> Logical Operator/1
  Q_dly/1 -> Logical Operator2/2
  Logical Operator2/1 -> Logical Operator/2
  Logical Operator/1 -> Q/1, Logical Operator3/1, Q_dly/1
  Logical Operator3/1 -> Q!/1
  Reset_b/1 -> Logical Operator1/1
  Set_b/1 -> Logical Operator3/2, Logical Operator2/1

== system Sanu_Lib/Tapped_Delay_Dynamic ==
  inp : Inport
  Arr_Length : Inport  Port=2  OutDataTypeStr=uint8
  Tapped_Delay : Stateflow chart  TreatAsAtomicUnit=on
  tapped_dly_out : UnitDelay  SampleTime=-1  HasFrameUpgradeWarning=on
      settings: AttributesFormatString=Init: %<InitialCondition>
  out : Outport
  wires:
  Tapped_Delay/1(out) -> tapped_dly_out/1
  tapped_dly_out/1 -> out/1
  inp/1 -> Tapped_Delay/1(inp)
  Arr_Length/1 -> Tapped_Delay/2(Arr_Length)

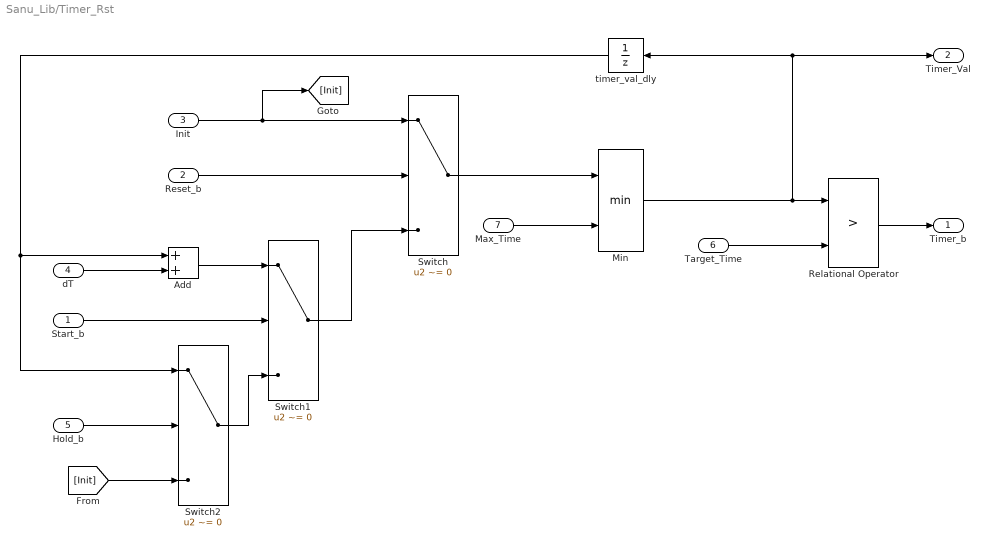
== system Sanu_Lib/Timer_Rst ==
  Start_b : Inport  OutDataTypeStr=boolean
  Reset_b : Inport  Port=2  OutDataTypeStr=boolean
  Init : Inport  Port=3
  dT : Inport  Port=4
  Hold_b : Inport  Port=5  OutDataTypeStr=boolean
  Target_Time : Inport  Port=6
  Max_Time : Inport  Port=7
  Add : Sum
  Min : MinMax  Inputs=2  InputSameDT=on
  Relational Operator : RelationalOperator  Operator=>  OutDataTypeStr=boolean  RndMeth=Simplest
  Switch : Switch  Criteria=u2 ~= 0  SaturateOnIntegerOverflow=off  InputSameDT=off
  Switch1 : Switch  Criteria=u2 ~= 0  SaturateOnIntegerOverflow=off  InputSameDT=off
  Switch2 : Switch  Criteria=u2 ~= 0  SaturateOnIntegerOverflow=off  InputSameDT=off
  timer_val_dly : UnitDelay  SampleTime=-1  HasFrameUpgradeWarning=on
  Timer_b : Outport
  Timer_Val : Outport  Port=2
  wires:
  Reset_b/1 -> Switch/2
  Init/1 -> [Init], Switch/1
  Start_b/1 -> Switch1/2
  Add/1 -> Switch1/1
  Switch/1 -> Min/1
  dT/1 -> Add/2
  Switch1/1 -> Switch/3
  Switch2/1 -> Switch1/3
  Hold_b/1 -> Switch2/2
  [Init] -> Switch2/3
  Max_Time/1 -> Min/2
  Target_Time/1 -> Relational Operator/2
  Relational Operator/1 -> Timer_b/1
  Min/1 -> Relational Operator/1, timer_val_dly/1, Timer_Val/1
  timer_val_dly/1 -> Switch2/1, Add/1

== system Sanu_Lib/falling_edge ==
  in_b : Inport  OutDataTypeStr=boolean
  Logical Operator1 : Logic  Operator=NOT  AllPortsSameDT=off  OutDataTypeStr=boolean
  calc_out_b : Logic  AllPortsSameDT=off  OutDataTypeStr=boolean
  in_b_dly : UnitDelay  InitialCondition=false  SampleTime=-1  HasFrameUpgradeWarning=on
      settings: AttributesFormatString=Init: %<InitialCondition>
  out_b : Outport
  wires:
  in_b/1 -> in_b_dly/1, Logical Operator1/1
  in_b_dly/1 -> calc_out_b/2
  calc_out_b/1 -> out_b/1
  Logical Operator1/1 -> calc_out_b/1

== system Sanu_Lib/rising_edge ==
  in_b : Inport  OutDataTypeStr=boolean
  Logical Operator1 : Logic  Operator=NOT  AllPortsSameDT=off  OutDataTypeStr=boolean
  calc_out_b : Logic  AllPortsSameDT=off  OutDataTypeStr=boolean
  in_b_dly : UnitDelay  InitialCondition=false  SampleTime=-1  HasFrameUpgradeWarning=on
      settings: AttributesFormatString=Init: %<InitialCondition>
  out_b : Outport
  wires:
  in_b/1 -> in_b_dly/1, calc_out_b/1
  in_b_dly/1 -> Logical Operator1/1
  Logical Operator1/1 -> calc_out_b/2
  calc_out_b/1 -> out_b/1

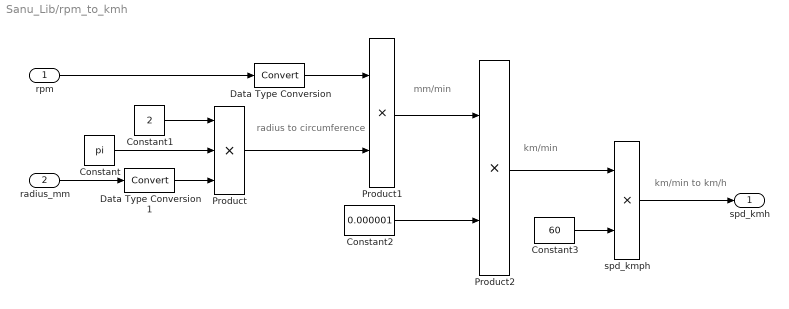
== system Sanu_Lib/rpm_to_kmh ==
  note: radius to circumference
  note: km/min
  note: km/min to km/h
  note: mm/min
  rpm : Inport
  radius_mm : Inport  Port=2
  Constant : Constant  Value=pi  OutDataTypeStr=single  SampleTime=-1
  Constant1 : Constant  Value=2  OutDataTypeStr=single  SampleTime=-1
  Constant2 : Constant  Value=0.000001  OutDataTypeStr=single  SampleTime=-1
  Constant3 : Constant  Value=60  OutDataTypeStr=single  SampleTime=-1
  Data Type Conversion : DataTypeConversion  SaturateOnIntegerOverflow=off  RndMeth=Floor
  Data Type Conversion1 : DataTypeConversion  SaturateOnIntegerOverflow=off  RndMeth=Floor
  Product : Product  Inputs=3
  Product1 : Product
  Product2 : Product
  spd_kmph : Product
  spd_kmh : Outport
  wires:
  Constant1/1 -> Product/1
  Constant/1 -> Product/2
  radius_mm/1 -> Data Type Conversion1/1
  Product/1 -> Product1/2
  Constant2/1 -> Product2/2
  Product1/1 -> Product2/1
  rpm/1 -> Data Type Conversion/1
  Product2/1 -> spd_kmph/1
  Constant3/1 -> spd_kmph/2
  spd_kmph/1 -> spd_kmh/1
  Data Type Conversion1/1 -> Product/3
  Data Type Conversion/1 -> Product1/1

== system Sanu_Lib/u16_to_u32_encoder ==
  ui16_low : Inport
  ui16_high : Inport  Port=2
  Bitwise OR : simulink/Logic and Bit Operations/Bitwise Operator  logicop=OR  UseBitMask=off  NumInputPorts=2  BitMask=bin2dec('11011001')  BitMaskRealWorld=Stored Integer
      settings: LibrarySourceBlock=|
      | simulink/Quick Insert/Logic and Bit
      | Operations/Bitwise OR
  Data Type Conversion : DataTypeConversion  OutDataTypeStr=uint32  SaturateOnIntegerOverflow=off  RndMeth=Floor
  Data Type Conversion1 : DataTypeConversion  OutDataTypeStr=uint32  SaturateOnIntegerOverflow=off  RndMeth=Floor
  Shift Arithmetic : ArithShift  BitShiftNumber=16  BitShiftDirection=Left
  ui32_val : Outport
  wires:
  Shift Arithmetic/1 -> Bitwise OR/1
  ui16_high/1 -> Data Type Conversion1/1
  ui16_low/1 -> Data Type Conversion/1
  Bitwise OR/1 -> ui32_val/1
  Data Type Conversion/1 -> Bitwise OR/2
  Data Type Conversion1/1 -> Shift Arithmetic/1

== system Sanu_Lib/u16_to_u8_cnv ==
  u16 : Inport
  Data Type Conversion : DataTypeConversion  OutDataTypeStr=uint16  SaturateOnIntegerOverflow=off  RndMeth=Floor
  Data Type Conversion1 : DataTypeConversion  OutDataTypeStr=uint8  SaturateOnIntegerOverflow=off  RndMeth=Floor
  Data Type Conversion2 : DataTypeConversion  OutDataTypeStr=uint8  SaturateOnIntegerOverflow=off  RndMeth=Floor
  Extract Bits : simulink/Logic and Bit Operations/Extract Bits  bitsToExtract=Upper half  numBits=8  bitIdxRange=[16 31]  outScalingMode=Treat bit field as an integer
  Extract Bits1 : simulink/Logic and Bit Operations/Extract Bits  bitsToExtract=Lower half  numBits=8  bitIdxRange=[0 15]  outScalingMode=Treat bit field as an integer
  u8_high : Outport
  u8_low : Outport  Port=2
  wires:
  Extract Bits/1 -> Data Type Conversion1/1
  Extract Bits1/1 -> Data Type Conversion2/1
  Data Type Conversion2/1 -> u8_low/1
  Data Type Conversion1/1 -> u8_high/1
  u16/1 -> Data Type Conversion/1
  Data Type Conversion/1 -> Extract Bits1/1, Extract Bits/1

== system Sanu_Lib/u32_to_u16_cnv ==
  u32 : Inport
  Data Type Conversion : DataTypeConversion  OutDataTypeStr=uint32  SaturateOnIntegerOverflow=off  RndMeth=Floor
  Data Type Conversion1 : DataTypeConversion  OutDataTypeStr=uint16  SaturateOnIntegerOverflow=off  RndMeth=Floor
  Data Type Conversion2 : DataTypeConversion  OutDataTypeStr=uint16  SaturateOnIntegerOverflow=off  RndMeth=Floor
  Extract Bits : simulink/Logic and Bit Operations/Extract Bits  bitsToExtract=Upper half  numBits=8  bitIdxRange=[16 31]  outScalingMode=Treat bit field as an integer
  Extract Bits1 : simulink/Logic and Bit Operations/Extract Bits  bitsToExtract=Lower half  numBits=8  bitIdxRange=[0 15]  outScalingMode=Treat bit field as an integer
  u16_high : Outport
  u16_low : Outport  Port=2
  wires:
  u32/1 -> Data Type Conversion/1
  Data Type Conversion/1 -> Extract Bits1/1, Extract Bits/1
  Extract Bits1/1 -> Data Type Conversion2/1
  Extract Bits/1 -> Data Type Conversion1/1
  Data Type Conversion1/1 -> u16_high/1
  Data Type Conversion2/1 -> u16_low/1

== stateflow chart Sanu_Lib/Counter_UI16 ==
  (default) -> (junction 1)
  (junction 1) -> (junction 3) [order 1] : [Reset_b == TRUE]
  (junction 1) -> (junction 5) [order 2]
  (junction 3) -> (junction 9) : {
      | Counter = 0;
      | Counter_b = FALSE;
      | }
  (junction 5) -> (junction 7) [order 1] : [Start_b == TRUE]
  (junction 7) -> (junction 13) [order 1] : [Counter >= Target_Cnt]
  (junction 5) -> (junction 20) [order 2]
  (junction 7) -> (junction 11) [order 2] : {
      | Counter++;
      | }
  (junction 13) -> (junction 15) : {
      | Counter_b = TRUE;
      | }
  (junction 20) -> (junction 22) [order 1] : [Hold_b == FALSE]
  (junction 20) -> (junction 24) [order 2]
  (junction 22) -> (junction 27) : {
      | Counter = 0;
      | Counter_b = FALSE;
      | }
  (junction 27) -> (junction 24)
  (junction 11) -> (junction 27)
  (junction 15) -> (junction 11)
  (junction 9) -> (junction 15)
  (junction 24) -> (junction 30)
  data: TRUE constant boolean =1; FALSE constant boolean =0; Start_b input boolean; Reset_b input boolean; Hold_b input boolean; Target_Cnt input uint16; Counter_b output boolean; Counter output uint16

== stateflow chart Sanu_Lib/Hysterisis_Logic/Hysterisis ==
  (default) -> (junction 1)
  (junction 1) -> (junction 3) [order 1] : [inp >= on_target + hyst]
  (junction 1) -> (junction 12) [order 2]
  (junction 3) -> (junction 5) : {
      | out_b = TRUE;
      | }
  (junction 12) -> (junction 14) [order 1] : [inp <= off_target - hyst]
  (junction 12) -> (junction 19) [order 2]
  (junction 14) -> (junction 16) : {
      | out_b = FALSE;
      | }
  (junction 16) -> (junction 19)
  (junction 5) -> (junction 16)
  (junction 19) -> (junction 22)
  data: TRUE constant boolean; FALSE constant boolean; inp input; on_target input; off_target input; out_b output boolean; hyst input

== stateflow chart Sanu_Lib/fibo_series_array_100_u8 ==
  note: n f(n)
      |
      | 0 0
      | 1 1
      | 2 1
      | 3 2
      | 4 3
      | 5 5
      | 6 8
      | 7 13
      | 8 21
      | 9 34
      | 10 55
      | 11 89
      | 12 144
      | 13 233
      | 14 377
      | 15 610
      | so on
  (default) -> (junction 25)
  (junction 25) -> (junction 26) [order 1] : [length <= 100]
  (junction 25) -> (junction 28) [order 2] : {idx = 100;}
  (junction 26) -> (junction 30) : {idx = length;}
  (junction 30) -> (junction 28)
  (junction 15) -> (junction 9) [order 1] : [i == 0]
  (junction 28) -> (junction 2)
  (junction 2) -> (junction 15) [order 1] : [i <= idx]
  (junction 15) -> (junction 8) [order 2]
  (junction 9) -> (junction 12) : {outp[i] = 0;}
  (junction 8) -> (junction 6) [order 1] : [i == 1 || i == 2]
  (junction 8) -> (junction 11) [order 2] : {
      | outp[i] = outp[i-1] + outp[i-2];
      | }
  (junction 6) -> (junction 19) : {
      | outp[i] = 1;
      | }
  (junction 11) -> (junction 2) : {
      | i++;
      | }
  (junction 2) -> (junction 14) [order 2]
  (junction 19) -> (junction 11)
  (junction 12) -> (junction 19)
  data: i local uint8; length input uint8; outp output single size=101; idx local uint8

== stateflow chart Sanu_Lib/temp_to_duty_cycle ==
  (default) -> (junction 1)
  (junction 1) -> (junction 3) [order 1] : [temp <= 0]
  (junction 1) -> (junction 13) [order 2]
  (junction 3) -> (junction 5) : {
      | pwm_duty_cycle = 0;
      | }
  (junction 13) -> (junction 15) [order 1] : [temp <= 40]
  (junction 13) -> (junction 19) [order 2]
  (junction 15) -> (junction 17) : {
      | pwm_duty_cycle = ...
      | (temp /40 ) * 40;
      | }
  (junction 19) -> (junction 21) [order 1] : [temp <= 60]
  (junction 19) -> (junction 25) [order 2]
  (junction 21) -> (junction 23) : {
      | pwm_duty_cycle = ...
      | 40 + (temp - 40 ) * 1.5;
      | }
  (junction 25) -> (junction 27) [order 1] : [temp <= 80]
  (junction 25) -> (junction 43) [order 2]
  (junction 27) -> (junction 29) : {
      | pwm_duty_cycle = ...
      | 70 + (temp - 60);
      | }
  (junction 43) -> (junction 45) [order 1] : [temp <= 90]
  (junction 43) -> (junction 31) [order 2] : {
      | pwm_duty_cycle = 100;
      | }
  (junction 45) -> (junction 47) : {
      | pwm_duty_cycle = ...
      | 90 + (temp - 80);
      | }
  (junction 47) -> (junction 31)
  (junction 29) -> (junction 47)
  (junction 23) -> (junction 29)
  (junction 17) -> (junction 23)
  (junction 5) -> (junction 17)
  (junction 31) -> (junction 38)
  data: temp input single; pwm_duty_cycle output uint8

== stateflow chart Sanu_Lib/Div_By_Zero_Handling ==
  (default) -> (junction 1)
  (junction 1) -> (junction 3) [order 1] : [denominator != 0]
  (junction 1) -> (junction 7) [order 2] : {
      | quotient = 0;
      | }
  (junction 3) -> (junction 5) : {
      | quotient = numerator / denominator;
      | }
  (junction 5) -> (junction 7)
  (junction 7) -> (junction 10)
  data: numerator input; denominator input; quotient output single

== stateflow chart Sanu_Lib/Set_Reset ==
  (default) -> (junction 1)
  (junction 1) -> (junction 3) [order 1] : [Reset_b == TRUE]
  (junction 1) -> (junction 7) [order 2]
  (junction 3) -> (junction 5) : {
      | Out_b = FALSE;
      | }
  (junction 7) -> (junction 9) [order 1] : [Set_b == TRUE]
  (junction 7) -> (junction 14) [order 2]
  (junction 9) -> (junction 11) : {
      | Out_b = TRUE;
      | }
  (junction 11) -> (junction 14)
  (junction 5) -> (junction 11)
  (junction 14) -> (junction 17)
  data: Set_b input boolean; Reset_b input boolean; Out_b output boolean; FALSE constant boolean =0; TRUE constant boolean =1

== stateflow chart Sanu_Lib/Tapped_Delay_Dynamic/Tapped_Delay ==
  note: Arr_Length max is 100
  (default) -> (junction 2)
  (junction 2) -> (junction 3) [order 1] : [i == 0]
  (junction 2) -> (junction 1) [order 2]
  (junction 3) -> (junction 6) : {
      | i++;
      | j = 0;
      | }
  (junction 1) -> (junction 23) [order 1] : [j < Arr_Length]
  (junction 1) -> (junction 8) [order 2] : {
      | j = 0;
      | }
  (junction 23) -> (junction 24) : {
      | out[j] = inp;
      | j++;
      | }
  (junction 8) -> (junction 17) [order 1] : [j == 0]
  (junction 8) -> (junction 25) [order 2]
  (junction 17) -> (junction 7) : {
      | out[j] = inp;
      | j++;
      | }
  (junction 7) -> (junction 25)
  (junction 24) -> (junction 7)
  (junction 6) -> (junction 24)
  (junction 25) -> (junction 9)
  data: inp input; i local uint8; out output size=100; Arr_Length input uint8 [0..100]; j local uint8
